simulink model "test_sim"  (Simulink 10.3)
settings: Solver=FixedStepAuto  StartTime=0.0  StopTime=5  FixedStep=0.00001  RelTol=1e-3  EnableMultiTasking=on
settings Model: Creator=ljk  LastModifiedBy=fu  ExtModeTrigMode=oneshot  ExtModeArmWhenConnect=off
settings OptimizationCC: BlockReduction=off  BooleanDataType=off
settings DebuggingCC: SaveWithParameterizedLinksMsg=none  SignalResolutionControl=TryResolveAllWithWarning  MultiTaskDSMMsg=warning  MultiTaskCondExecSysMsg=none
settings HardwareCC: TargetUnknown=on

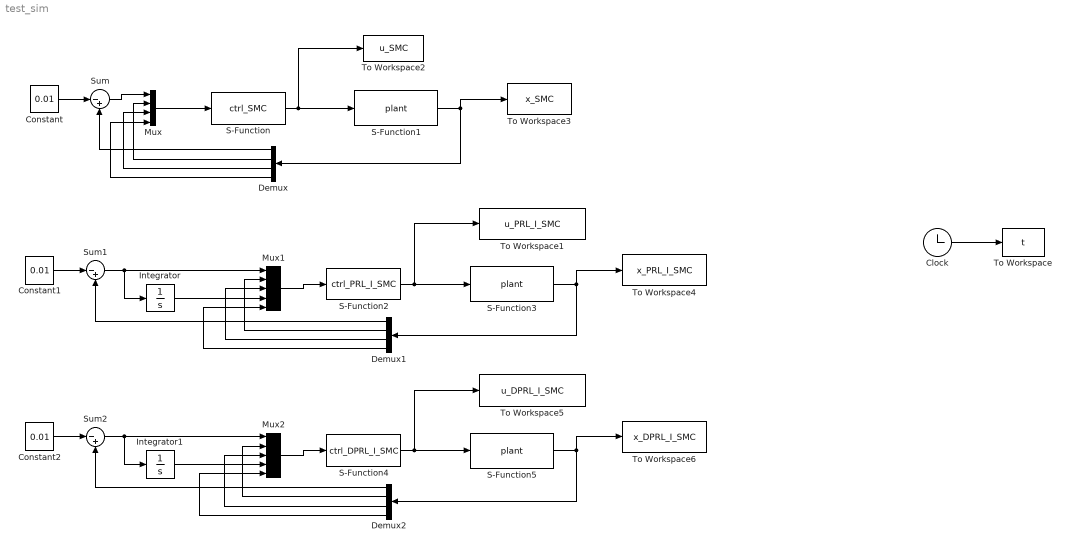
== system test_sim ==
  Clock : Clock
  Constant : Constant  Value=0.01  VectorParams1D=off
  Constant1 : Constant  Value=0.01  VectorParams1D=off
  Constant2 : Constant  Value=0.01  VectorParams1D=off
  Demux : Demux
  Demux1 : Demux
  Demux2 : Demux
  Integrator : Integrator
  Integrator1 : Integrator
  Mux : Mux
  Mux1 : Mux  Inputs=5
  Mux2 : Mux  Inputs=5
  S-Function : S-Function  FunctionName=ctrl_SMC  SFunctionDeploymentMode=off  EnableBusSupport=off
  S-Function1 : S-Function  FunctionName=plant  SFunctionDeploymentMode=off  EnableBusSupport=off
  S-Function2 : S-Function  FunctionName=ctrl_PRL_I_SMC  SFunctionDeploymentMode=off  EnableBusSupport=off
  S-Function3 : S-Function  FunctionName=plant  SFunctionDeploymentMode=off  EnableBusSupport=off
  S-Function4 : S-Function  FunctionName=ctrl_DPRL_I_SMC  SFunctionDeploymentMode=off  EnableBusSupport=off
  S-Function5 : S-Function  FunctionName=plant  SFunctionDeploymentMode=off  EnableBusSupport=off
  Sum : Sum  Inputs=|-+
  Sum1 : Sum  Inputs=|-+
  Sum2 : Sum  Inputs=|-+
  To Workspace : ToWorkspace  VariableName=t  SampleTime=-1
  To Workspace1 : ToWorkspace  VariableName=u_PRL_I_SMC  SampleTime=-1
  To Workspace2 : ToWorkspace  VariableName=u_SMC  SampleTime=-1
  To Workspace3 : ToWorkspace  VariableName=x_SMC  SampleTime=-1
  To Workspace4 : ToWorkspace  VariableName=x_PRL_I_SMC  SampleTime=-1
  To Workspace5 : ToWorkspace  VariableName=u_DPRL_I_SMC  SampleTime=-1
  To Workspace6 : ToWorkspace  VariableName=x_DPRL_I_SMC  SampleTime=-1
  wires:
  S-Function/1 -> To Workspace2/1, S-Function1/1
  Clock/1 -> To Workspace/1
  S-Function1/1 -> To Workspace3/1, Demux/1
  Constant/1 -> Sum/1
  Demux/1 -> Sum/2
  Sum/1 -> Mux/1
  Mux/1 -> S-Function/1
  Demux/2 -> Mux/2
  Demux/3 -> Mux/3
  Demux1/3 -> Mux1/3
  Mux1/1 -> S-Function2/1
  Constant1/1 -> Sum1/1
  Demux1/1 -> Sum1/2
  Sum1/1 -> Integrator/1, Mux1/1
  S-Function3/1 -> To Workspace4/1, Demux1/1
  S-Function2/1 -> To Workspace1/1, S-Function3/1
  Demux1/2 -> Mux1/2
  Integrator/1 -> Mux1/4
  Integrator1/1 -> Mux2/4
  Sum2/1 -> Integrator1/1, Mux2/1
  Demux2/3 -> Mux2/3
  Demux2/1 -> Sum2/2
  Demux2/2 -> Mux2/2
  Mux2/1 -> S-Function4/1
  S-Function5/1 -> To Workspace6/1, Demux2/1
  S-Function4/1 -> To Workspace5/1, S-Function5/1
  Constant2/1 -> Sum2/1
  Demux1/4 -> Mux1/5
  Demux2/4 -> Mux2/5
  Demux/4 -> Mux/4
